simulink model "fstd_avion"  (R2020b)
settings: Solver=VariableStepAuto  StartTime=0.0  StopTime=10.0  RelTol=1e-3
values from neighbouring files (symbols this model uses):
  plant = ss(a,b,c,d)    [data_avion_lat.m]
libraries: cstblocks x2
settings Model: Creator=d.alazard  LastModifiedBy=d.alazard
settings DataIOCC: ReturnWorkspaceOutputs=off
settings DebuggingCC: ArithmeticOperatorsInVariantConditions=warning
settings SFSimCC: CustomCodeUndefinedFunction=UseInterfaceOnly

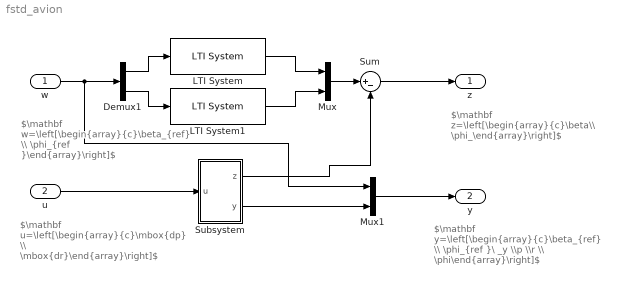
== system fstd_avion ==
  note: $\mathbf w=\left[\begin{array}{c}\beta_{ref} \\ \phi_{ref }\end{array}\right]$
  note: $\mathbf u=\left[\begin{array}{c}\mbox{dp} \\ \mbox{dr}\end{array}\right]$
  note: $\mathbf z=\left[\begin{array}{c}\beta\\ \phi_\end{array}\right]$
  note: $\mathbf y=\left[\begin{array}{c}\beta_{ref} \\ \phi_{ref }\\n_y \\p \\r \\ \phi\end{array}\right]$
  w : Inport  PortDimensions=2
  u : Inport  Port=2
  Demux1 : Demux  Outputs=2
  LTI System : cstblocks/LTI System  sys=F1  IC=[]
  LTI System1 : cstblocks/LTI System  sys=F2  IC=[]
  Mux : Mux  Inputs=2
  Mux1 : Mux  Inputs=[2 4]
  Subsystem : Subsystem
  Sum : Sum  Inputs=|+-
  z : Outport  VectorParamsAs1DForOutWhenUnconnected=off
  y : Outport  Port=2  VectorParamsAs1DForOutWhenUnconnected=off
  wires:
  u/1 -> Subsystem/1(u)
  LTI System/1 -> Mux/1
  LTI System1/1 -> Mux/2
  Demux1/1 -> LTI System/1
  Demux1/2 -> LTI System1/1
  w/1 -> Mux1/1, Demux1/1
  Subsystem/2(y) -> Mux1/2
  Mux1/1 -> y/1
  Mux/1 -> Sum/1
  Sum/1 -> z/1
  Subsystem/1(z) -> Sum/2

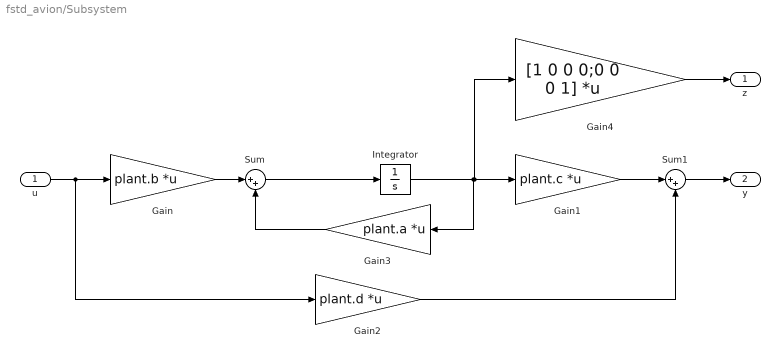
== system fstd_avion/Subsystem ==
  u : Inport
  Gain : Gain  Gain=plant.b  Multiplication=Matrix(K*u) (u vector)
  Gain1 : Gain  Gain=plant.c  Multiplication=Matrix(K*u) (u vector)
  Gain2 : Gain  Gain=plant.d  Multiplication=Matrix(K*u) (u vector)
  Gain3 : Gain  Gain=plant.a  Multiplication=Matrix(K*u) (u vector)
  Gain4 : Gain  Gain=[1 0 0 0;0 0 0 1]  Multiplication=Matrix(K*u) (u vector)
  Integrator : Integrator
  Sum : Sum  Inputs=|++
  Sum1 : Sum  Inputs=|++
  z : Outport  VectorParamsAs1DForOutWhenUnconnected=off
  y : Outport  Port=2  VectorParamsAs1DForOutWhenUnconnected=off
  wires:
  Gain/1 -> Sum/1
  u/1 -> Gain2/1, Gain/1
  Gain2/1 -> Sum1/2
  Gain3/1 -> Sum/2
  Gain4/1 -> z/1
  Sum/1 -> Integrator/1
  Sum1/1 -> y/1
  Gain1/1 -> Sum1/1
  Integrator/1 -> Gain3/1, Gain4/1, Gain1/1
